simulink model "MCU_CmdTransV4"  (R2022b)
settings: Solver=FixedStepDiscrete  StartTime=0.0  StopTime=10.0  FixedStep=0.001  RelTol=1e-3
undefined symbols (not defined in the file or in its folder): ANALOG, cAgeingMode, cCurrentLoopMode, cNoneMode, cParaRecogMode, cSingleBoardMode, cSpeedLoopMode, cTorqueLoopMode, cVvvfOpenMode, FAULT, ParamCfg_CommandSource_u16, ParamCfg_MaxSpeed_u16, ParamCfg_MaxTorque_u16, ParamCfg_Spdouttype_u16, ParamCfg_Vc1Enable_u16, POWER_ON, STANDBY, TESTBED, VEHICLE
libraries: simulink x8
(part 2 of 2)

== stateflow chart MCU_CmdTransV4/Can2Model_2ms/CAN2Source/状态机备份/Chart1 ==
  (default) -> (junction 422)
  (junction 422) -> (junction 647) [order 1] : [ModeCmd == cNoneMode ]
      | {
      | WorkCmdSourceRunCmd = 0;
      | WorkCmdSourceDisChargeCmd = 0;
      | WorkCmdSourceModeCmd = cNoneMode;
      | WorkCmdSourceTorqueCmd = 0;
      | WorkCmdSourceSpeedCmd = 0;
      | WorkCmdSourceCurrentCmd = 0;
      | WorkCmdSourceThetaCmd = 0;
      | WorkCmdSourceIsdCmd = 0;
      | WorkCmdSourceIsqCmd = 0;
      | WorkCmdSourceFreqCmd = 0;
      | }
  (junction 422) -> (junction 647) [order 2]
  (junction 647) -> (junction 565)
  (junction 565) -> (junction 566) [order 1] : [ModeCmd==cTorqueLoopMode || FaultCheck_LostPhaseFaultFlg ==1]
  (junction 565) -> (junction 558) [order 2]
  (junction 566) -> (junction 653) : {WorkingModeSelect = cTorqueLoopMode;
      | WorkCmdSourceTorqueCmd = TorqueCmd;}
  (junction 653) -> (junction 563) [order 1] : [FaultCheck_LostPhaseFaultFlg ==1]{WorkCmdSourceRunCmd = 1}
  (junction 653) -> (junction 563) [order 2] : {WorkCmdSourceRunCmd = RunCmd;}
  (junction 563) -> (junction 561)
  (junction 558) -> (junction 562) [order 1] : [ModeCmd ==cSpeedLoopMode ]
  (junction 558) -> (junction 576) [order 2]
  (junction 562) -> (junction 564) : {WorkingModeSelect = cSpeedLoopMode;
      | WorkCmdSourceRunCmd = RunCmd;
      | WorkCmdSourceSpeedCmd = SpeedCmd;}
  (junction 560) -> (junction 561) [order 1] : [ModeSelectBefore ~= cSpeedLoopMode]{SpeedCtrl_SpeedCmdFilter = SpeedCal_speed2ms}
  (junction 564) -> (junction 560)
  (junction 560) -> (junction 561) [order 2]
  (junction 561) -> (junction 568)
  (junction 576) -> (junction 570) [order 1] : [ModeCmd ==cCurrentLoopMode ]
  (junction 576) -> (junction 569) [order 2]
  (junction 570) -> (junction 579) : {WorkingModeSelect = cCurrentLoopMode;
      | WorkCmdSourceRunCmd = RunCmd;}
  (junction 579) -> (junction 567) [order 1] : [CurrentPolarCoordinatesFlg ==1]
  (junction 579) -> (junction 573) [order 2] : {WorkCmdSourceIsdCmd = IsdCmd;
      | WorkCmdSourceIsqCmd = IsqCmd}
  (junction 567) -> (junction 575) : {WorkCmdSourceCurrentCmd = CurrentCmd;
      | WorkCmdSourceThetaCmd = ThetaCmd;}
  (junction 575) -> (junction 573)
  (junction 573) -> (junction 572)
  (junction 572) -> (junction 568)
  (junction 568) -> (junction 574)
  (junction 569) -> (junction 571) [order 1] : [ModeCmd ==cVvvfOpenMode ]
  (junction 569) -> (junction 578) [order 2]
  (junction 571) -> (junction 577) : {WorkingModeSelect = cVvvfOpenMode;
      | WorkCmdSourceRunCmd = RunCmd;
      | WorkCmdSourceFreqCmd = FreqCmd;}
  (junction 577) -> (junction 574)
  (junction 574) -> (junction 581)
  (junction 578) -> (junction 586) [order 1] : [ModeCmd ==cParaRecogMode ]
  (junction 578) -> (junction 590) [order 2]
  (junction 586) -> (junction 597) : {WorkingModeSelect = cParaRecogMode;
      | WorkCmdSourceRunCmd = RunCmd;}
  (junction 597) -> (junction 581)
  (junction 581) -> (junction 585)
  (junction 590) -> (junction 587) [order 1] : [ModeCmd ==cSingleBoardMode ]
  (junction 590) -> (junction 582) [order 2]
  (junction 587) -> (junction 583) : {WorkingModeSelect = cSingleBoardMode;
      | WorkCmdSourceRunCmd = RunCmd;}
  (junction 583) -> (junction 585)
  (junction 585) -> (junction 592)
  (junction 582) -> (junction 591) [order 1] : [ModeCmd ==cAgeingMode ]
  (junction 582) -> (junction 598) [order 2]
  (junction 591) -> (junction 596) : {WorkingModeSelect = cAgeingMode;
      | WorkCmdSourceRunCmd = RunCmd;
      | WorkCmdSourceCurrentCmd = CurrentCmd;
      | WorkCmdSourceThetaCmd = ThetaCmd;
      | WorkCmdSourceFreqCmd = FreqCmd;}
  (junction 596) -> (junction 592)
  (junction 592) -> (junction 595)
  (junction 598) -> (junction 599) [order 1] : [ModeCmd ==cNoneMode ]
  (junction 598) -> (junction 588) [order 2] : {WorkingModeSelect = cNoneMode;
      | WorkCmdSourceRunCmd = 0;
      | WorkCmdSourceDisChargeCmd = 0;
      | WorkCmdSourceModeCmd = cNoneMode;
      | WorkCmdSourceTorqueCmd = 0;
      | WorkCmdSourceSpeedCmd = 0;
      | WorkCmdSourceCurrentCmd = 0;
      | WorkCmdSourceThetaCmd = 0;
      | WorkCmdSourceIsdCmd = 0;
      | WorkCmdSourceIsqCmd = 0;
      | WorkCmdSourceFreqCmd = 0;}
  (junction 599) -> (junction 584) : {WorkingModeSelect = cNoneMode;
      | WorkCmdSourceRunCmd = RunCmd;}
  (junction 584) -> (junction 595)
  (junction 595) -> (junction 593)
  (junction 593) -> (junction 588)
  (junction 588) -> (junction 644) [order 1] : [LsDepFlg == 1]{WorkCmdSourceTorqueCmd=0}
  (junction 588) -> (junction 644) [order 2]
  (junction 644) -> (junction 637)
  (junction 637) -> (junction 643) [order 2] : [ActDisChargeStd == 1]...
      | {WorkCmdSourceRunCmd = 1;
      | WorkCmdSourceModeCmd = cCurrentLoopMode;
      | WorkCmdSourceIsdCmd = ActDisChargeCurr;
      | WorkCmdSourceIsqCmd = 0;
      | CurrentPolarCoordinates =0;}
  (junction 637) -> (junction 643) [order 1]
  (junction 643) -> (junction 645)
  (junction 645) -> (junction 589)
  (junction 589) -> (junction 600) [order 1] : [ZeroTorqueFlag == 1]
      | {WorkingModeSelect = cTorqueLoopMode;
      | WorkCmdSourceRunCmd = RunCmd;
      | WorkCmdSourceTorqueCmd = 0;}
  (junction 589) -> (junction 600) [order 2]
  (junction 600) -> (junction 594) [order 1] : [ClosePWMFlg == 1 ]
      | {
      | WorkCmdSourceRunCmd = 0;
      | WorkCmdSourceDisChargeCmd = 0;
      | WorkCmdSourceModeCmd = cNoneMode;
      | WorkCmdSourceTorqueCmd = 0;
      | WorkCmdSourceSpeedCmd = 0;
      | WorkCmdSourceCurrentCmd = 0;
      | WorkCmdSourceThetaCmd = 0;
      | WorkCmdSourceIsdCmd = 0;
      | WorkCmdSourceIsqCmd = 0;
      | WorkCmdSourceFreqCmd = 0;
      | }
  (junction 600) -> (junction 594) [order 2]
  (junction 594) -> (junction 661)
  data: RunCmd input; WorkCmdSourceRunCmd output uint16 =0; WorkCmdSourceDisChargeCmd output uint16 =0; WorkCmdSourceModeCmd output uint16 =0; WorkCmdSourceTorqueCmd output single =0; WorkCmdSourceSpeedCmd output single =0; WorkCmdSourceCurrentCmd output single =0; WorkCmdSourceThetaCmd output single =0; WorkCmdSourceIsdCmd output single =0; WorkCmdSourceIsqCmd output single =0; WorkCmdSourceFreqCmd output single =0; DisChargeCmd input; ModeCmd input; TorqueCmd input; SpeedCmd input; CurrentCmd input; ThetaCmd input; IsdCmd input; IsqCmd input; FreqCmd input; ActDisChargeStd input; ActDisChargeCurr input; FaultCheck_LostPhaseFaultFlg input; LsDepFlg input; cTorqueLoopMode parameter; cCurrentLoopMode parameter; CurrentPolarCoordinates output uint16 =0; VEHICLE parameter; TESTBED parameter; ANALOG parameter; cAgeingMode parameter; cNoneMode parameter; cParaRecogMode parameter; cSingleBoardMode parameter; cSpeedLoopMode parameter; cVvvfOpenMode parameter; WorkingModeSelect output double; ModeSelectBefore input; SpeedCal_speed2ms input; SpeedCtrl_SpeedCmdFilter local double; ZeroTorqueFlag input; CurrentPolarCoordinatesFlg input; ClosePWMFlg input

== stateflow chart MCU_CmdTransV4/TaskCmdCal_1ms/Cmd2Task/Cmd2Task ==
  note: 当前转速可以关管
  (default) -> (junction 18)
  (junction 18) -> (junction 20) [order 1] : [WorkState_ModeSelect ==cTorqueLoopMode]
  (junction 18) -> (junction 50) [order 2]
  (junction 20) -> (junction 22) : {
      | WorkCmdTaskRunCmd = WorkCmdRunCmd;
      | WorkCmdTaskTorqueCmd = WorkCmdTorqueCmd;
      | }
  (junction 28) -> (junction 32) [order 1] : [(SpeedCal_HighSpdZeroTrqFlg == 0)&&(TorqeCtrl_TorqueCmdFilterAbs<0.001) && (WorkCmdTaskTorqueCmd < 0.001)]{WorkCmdTaskRunCmd = STOP}
  (junction 22) -> (junction 25) [order 1] : [WorkCmdTaskTorqueCmd > 0]{SpeedCmdDir =1}
  (junction 22) -> (junction 25) [order 2] : {SpeedCmdDir = -1}
  (junction 25) -> (junction 28) : {WorkCmdTaskSpeedCmd = ParamCfg_MaxSpeed_u16 * SpeedCmdDir}
  (junction 28) -> (junction 32) [order 2]
  (junction 32) -> (junction 58)
  (junction 50) -> (junction 52) [order 1] : [WorkState_ModeSelect == cSpeedLoopMode]
  (junction 50) -> (junction 61) [order 2]
  (junction 52) -> (junction 54) : {WorkCmdTaskRunCmd = WorkCmdRunCmd;
      | WorkCmdTaskSpeedCmd = WorkCmdSpeedCmd;
      | WorkCmdTaskTorqueCmd = (ParamCfg_MaxTorque_u16 * 0.1)}
  (junction 54) -> (junction 58)
  (junction 58) -> (junction 67)
  (junction 61) -> (junction 63) [order 1] : [WorkState_ModeSelect == cCurrentLoopMode ]
  (junction 61) -> (junction 78) [order 2]
  (junction 63) -> (junction 65) : {WorkCmdTaskRunCmd = WorkCmdRunCmd}
  (junction 71) -> (junction 67) [order 1] : [(CurrentPolar == 1)&&ParamCfg_CommandSource_u16 == TESTBED]...
      | {WorkCmdTaskCurrentCmd = WorkCmdCurrentCmd;
      | WorkCmdTaskThetaCmd = WorkCmdThetaCmd;
      | WorkCmdTaskIsdCmd = WorkCmdTaskCurrentCmd * cos(WorkCmdTaskThetaCmd)*(-1)
      | WorkCmdTaskIsqCmd = WorkCmdTaskCurrentCmd * sin(WorkCmdTaskThetaCmd)
      | }
  (junction 71) -> (junction 67) [order 2] : {WorkCmdTaskIsdCmd = WorkCmdIsdCmd;
      | WorkCmdTaskIsqCmd = WorkCmdIsqCmd}
  (junction 65) -> (junction 71)
  (junction 67) -> (junction 85)
  (junction 78) -> (junction 80) [order 1] : [WorkState_ModeSelect == cVvvfOpenMode ]
  (junction 78) -> (junction 88) [order 2]
  (junction 80) -> (junction 83) : {WorkCmdTaskRunCmd = WorkCmdRunCmd;
      | WorkCmdTaskIsdCmd = WorkCmdIsdCmd;
      | WorkCmdTaskIsqCmd = WorkCmdIsqCmd;
      | WorkCmdTaskFreqCmd = WorkCmdFreqCmd;
      | }
  (junction 83) -> (junction 85)
  (junction 85) -> (junction 95)
  (junction 88) -> (junction 90) [order 1] : [WorkState_ModeSelect == cParaRecogMode ]
  (junction 88) -> (junction 98) [order 2]
  (junction 90) -> (junction 93) : {WorkCmdTaskRunCmd = WorkCmdRunCmd;
      | WorkCmdTaskRunCmd = WorkCmdRunCmd;
      | WorkCmdTaskIsdCmd = WorkCmdIsdCmd;
      | WorkCmdTaskIsqCmd = WorkCmdIsqCmd}
  (junction 93) -> (junction 95)
  (junction 95) -> (junction 105)
  (junction 98) -> (junction 100) [order 1] : [WorkState_ModeSelect == cSingleBoardMode ]
  (junction 98) -> (junction 108) [order 2]
  (junction 100) -> (junction 103) : {WorkCmdTaskRunCmd = WorkCmdRunCmd}
  (junction 103) -> (junction 105)
  (junction 105) -> (junction 125)
  (junction 108) -> (junction 110) [order 1] : [WorkState_ModeSelect == cAgeingMode ]
  (junction 108) -> (junction 112) [order 2]
  (junction 110) -> (junction 118) : {WorkCmdTaskRunCmd     = WorkCmdRunCmd;
      |  WorkCmdTaskCurrentCmd = (WorkCmdCurrentCmd);
      | WorkCmdTaskThetaCmd   = WorkCmdThetaCmd;
      |  WorkCmdTaskIsdCmd     = (WorkCmdTaskCurrentCmd * cos(WorkCmdTaskThetaCmd*2*PI));
      |  WorkCmdTaskIsqCmd     = (WorkCmdTaskCurrentCmd * sin(WorkCmdTaskThetaCmd*2*PI));
      |   WorkCmdTaskFreqCmd    = WorkCmdFreqCmd;}
  (junction 118) -> (junction 125)
  (junction 125) -> (junction 122)
  (junction 112) -> (junction 114) [order 1] : [WorkState_ModeSelect == cNoneMode ]
  (junction 112) -> (junction 129) [order 2]
  (junction 114) -> (junction 120) : {WorkCmdTaskRunCmd = STOP}
  (junction 120) -> (junction 122)
  (junction 122) -> (junction 131)
  (junction 131) -> (junction 129)
  (junction 129) -> (junction 134)
  data: WorkCmdIsdCmd input; WorkState_ModeSelect input; WorkCmdRunCmd input; WorkCmdTorqueCmd input; WorkCmdSpeedCmd input; WorkCmdCurrentCmd input; WorkCmdThetaCmd input; WorkCmdIsqCmd input; WorkCmdFreqCmd input; WorkCmdTaskRunCmd output uint16 =0; WorkCmdTaskTorqueCmd output single =0; WorkCmdTaskSpeedCmd output single =0; WorkCmdTaskCurrentCmd output single =0; WorkCmdTaskThetaCmd output single =0; WorkCmdTaskIsdCmd output single =0; WorkCmdTaskIsqCmd output single =0; WorkCmdTaskFreqCmd output single =0; cTorqueLoopMode parameter; SpeedCmdDir output int16 =1; SpeedCal_HighSpdZeroTrqFlg input; TorqeCtrl_TorqueCmdFilterAbs input; ParamCfg_MaxSpeed_u16 parameter; STOP constant uint16 =0; cSpeedLoopMode parameter; cCurrentLoopMode parameter; ParamCfg_MaxTorque_u16 parameter; CurrentPolar input; ParamCfg_CommandSource_u16 parameter; TESTBED parameter; cVvvfOpenMode parameter; cParaRecogMode parameter; cSingleBoardMode parameter; cAgeingMode parameter; cNoneMode parameter; PI constant single =3.141592

== stateflow chart MCU_CmdTransV4/Can2Model_2ms/CAN2Source/CANTransChart ==
  (default) -> (junction 422)
  (junction 422) -> (junction 647) [order 1] : [ModeCmd == cNoneMode ]
      | {
      | WorkCmdSourceRunCmd = 0;
      | WorkCmdSourceDisChargeCmd = 0;
      | WorkCmdSourceModeCmd = cNoneMode;
      | WorkCmdSourceTorqueCmd = 0;
      | WorkCmdSourceSpeedCmd = 0;
      | WorkCmdSourceCurrentCmd = 0;
      | WorkCmdSourceThetaCmd = 0;
      | WorkCmdSourceIsdCmd = 0;
      | WorkCmdSourceIsqCmd = 0;
      | WorkCmdSourceFreqCmd = 0;
      | }
  (junction 422) -> (junction 647) [order 2]
  (junction 647) -> (junction 565)
  (junction 565) -> (junction 566) [order 1] : [ModeCmd==cTorqueLoopMode || FaultCheck_LostPhaseFaultFlg ==1 || ZeroTorqueFlag == 1]
  (junction 565) -> (junction 558) [order 2]
  (junction 566) -> (junction 664) : {WorkingModeSelect = cTorqueLoopMode;}
  (junction 667) -> (junction 563) [order 1] : [ZeroTorqueFlag == 1]{WorkCmdSourceTorqueCmd = 0}
  (junction 664) -> (junction 667) [order 1] : [FaultCheck_LostPhaseFaultFlg ==1]{WorkCmdSourceRunCmd = 1}
  (junction 664) -> (junction 667) [order 2] : {WorkCmdSourceRunCmd = RunCmd;}
  (junction 667) -> (junction 563) [order 2] : {WorkCmdSourceTorqueCmd = TorqueCmd;}
  (junction 563) -> (junction 561)
  (junction 558) -> (junction 562) [order 1] : [ModeCmd ==cSpeedLoopMode ]
  (junction 558) -> (junction 576) [order 2]
  (junction 562) -> (junction 564) : {WorkingModeSelect = cSpeedLoopMode;
      | WorkCmdSourceRunCmd = RunCmd;
      | WorkCmdSourceSpeedCmd = SpeedCmd;}
  (junction 560) -> (junction 561) [order 1] : [ModeSelectBefore ~= cSpeedLoopMode]{SpeedCtrl_SpeedCmdFilter = SpeedCal_speed2ms}
  (junction 564) -> (junction 560)
  (junction 560) -> (junction 561) [order 2]
  (junction 561) -> (junction 568)
  (junction 576) -> (junction 570) [order 1] : [ModeCmd ==cCurrentLoopMode ]
  (junction 576) -> (junction 569) [order 2]
  (junction 570) -> (junction 579) : {WorkingModeSelect = cCurrentLoopMode;
      | WorkCmdSourceRunCmd = RunCmd;}
  (junction 579) -> (junction 567) [order 1] : [CurrentPolarCoordinatesFlg ==1]
  (junction 579) -> (junction 573) [order 2] : {WorkCmdSourceIsdCmd = IsdCmd;
      | WorkCmdSourceIsqCmd = IsqCmd}
  (junction 567) -> (junction 575) : {WorkCmdSourceCurrentCmd = CurrentCmd;
      | WorkCmdSourceThetaCmd = ThetaCmd;}
  (junction 575) -> (junction 573)
  (junction 573) -> (junction 572)
  (junction 572) -> (junction 568)
  (junction 568) -> (junction 574)
  (junction 569) -> (junction 571) [order 1] : [ModeCmd ==cVvvfOpenMode ]
  (junction 569) -> (junction 578) [order 2]
  (junction 571) -> (junction 577) : {WorkingModeSelect = cVvvfOpenMode;
      | WorkCmdSourceRunCmd = RunCmd;
      | WorkCmdSourceFreqCmd = FreqCmd;}
  (junction 577) -> (junction 574)
  (junction 574) -> (junction 581)
  (junction 578) -> (junction 586) [order 1] : [ModeCmd ==cParaRecogMode ]
  (junction 578) -> (junction 590) [order 2]
  (junction 586) -> (junction 597) : {WorkingModeSelect = cParaRecogMode;
      | WorkCmdSourceRunCmd = RunCmd;}
  (junction 597) -> (junction 581)
  (junction 581) -> (junction 585)
  (junction 590) -> (junction 587) [order 1] : [ModeCmd ==cSingleBoardMode ]
  (junction 590) -> (junction 582) [order 2]
  (junction 587) -> (junction 583) : {WorkingModeSelect = cSingleBoardMode;
      | WorkCmdSourceRunCmd = RunCmd;}
  (junction 583) -> (junction 585)
  (junction 585) -> (junction 592)
  (junction 582) -> (junction 591) [order 1] : [ModeCmd ==cAgeingMode ]
  (junction 582) -> (junction 598) [order 2]
  (junction 591) -> (junction 596) : {WorkingModeSelect = cAgeingMode;
      | WorkCmdSourceRunCmd = RunCmd;
      | WorkCmdSourceCurrentCmd = CurrentCmd;
      | WorkCmdSourceThetaCmd = ThetaCmd;
      | WorkCmdSourceFreqCmd = FreqCmd;}
  (junction 596) -> (junction 592)
  (junction 592) -> (junction 595)
  (junction 598) -> (junction 599) [order 1] : [ModeCmd ==cNoneMode ]
  (junction 598) -> (junction 588) [order 2] : {WorkingModeSelect = cNoneMode;
      | WorkCmdSourceRunCmd = 0;
      | WorkCmdSourceDisChargeCmd = 0;
      | WorkCmdSourceModeCmd = cNoneMode;
      | WorkCmdSourceTorqueCmd = 0;
      | WorkCmdSourceSpeedCmd = 0;
      | WorkCmdSourceCurrentCmd = 0;
      | WorkCmdSourceThetaCmd = 0;
      | WorkCmdSourceIsdCmd = 0;
      | WorkCmdSourceIsqCmd = 0;
      | WorkCmdSourceFreqCmd = 0;}
  (junction 599) -> (junction 584) : {WorkingModeSelect = cNoneMode;
      | WorkCmdSourceRunCmd = RunCmd;}
  (junction 584) -> (junction 595)
  (junction 595) -> (junction 593)
  (junction 593) -> (junction 588)
  (junction 588) -> (junction 644) [order 1] : [LsDepFlg == 1]{WorkCmdSourceTorqueCmd=0}
  (junction 588) -> (junction 644) [order 2]
  (junction 644) -> (junction 637)
  (junction 637) -> (junction 643) [order 1] : [ActDisChargeStd == 1]...
      | {WorkCmdSourceRunCmd = 1;
      | WorkCmdSourceModeCmd = cCurrentLoopMode;
      | WorkCmdSourceIsdCmd = ActDisChargeCurr;
      | WorkCmdSourceIsqCmd = 0;
      | CurrentPolarCoordinates =0;}
  (junction 637) -> (junction 643) [order 2]
  (junction 643) -> (junction 600)
  (junction 600) -> (junction 594) [order 1] : [ClosePWMFlg == 1 ]
      | {
      | WorkCmdSourceRunCmd = 0;
      | WorkCmdSourceDisChargeCmd = 0;
      | WorkCmdSourceModeCmd = cNoneMode;
      | WorkCmdSourceTorqueCmd = 0;
      | WorkCmdSourceSpeedCmd = 0;
      | WorkCmdSourceCurrentCmd = 0;
      | WorkCmdSourceThetaCmd = 0;
      | WorkCmdSourceIsdCmd = 0;
      | WorkCmdSourceIsqCmd = 0;
      | WorkCmdSourceFreqCmd = 0;
      | }
  (junction 600) -> (junction 594) [order 2]
  (junction 594) -> (junction 661)
  data: RunCmd input; WorkCmdSourceRunCmd output uint16 =0; WorkCmdSourceDisChargeCmd output uint16 =0; WorkCmdSourceModeCmd output uint16 =0; WorkCmdSourceTorqueCmd output single =0; WorkCmdSourceSpeedCmd output single =0; WorkCmdSourceCurrentCmd output single =0; WorkCmdSourceThetaCmd output single =0; WorkCmdSourceIsdCmd output single =0; WorkCmdSourceIsqCmd output single =0; WorkCmdSourceFreqCmd output single =0; DisChargeCmd input; ModeCmd input; TorqueCmd input; SpeedCmd input; CurrentCmd input; ThetaCmd input; IsdCmd input; IsqCmd input; FreqCmd input; ActDisChargeStd input; ActDisChargeCurr input; FaultCheck_LostPhaseFaultFlg input; LsDepFlg input; cTorqueLoopMode parameter; cCurrentLoopMode parameter; CurrentPolarCoordinates output uint16 =0; VEHICLE parameter; TESTBED parameter; ANALOG parameter; cAgeingMode parameter; cNoneMode parameter; cParaRecogMode parameter; cSingleBoardMode parameter; cSpeedLoopMode parameter; cVvvfOpenMode parameter; WorkingModeSelect output uint16 =cNoneMode; ModeSelectBefore input; SpeedCal_speed2ms input; SpeedCtrl_SpeedCmdFilter local double; ZeroTorqueFlag input; CurrentPolarCoordinatesFlg input; ClosePWMFlg input
